simulink model "exercise_5_1"  (R2024a)
settings: Solver=VariableStepDiscrete  StartTime=0.0  StopTime=inf  RelTol=1e-3  EnableMultiTasking=on
libraries: simulink_extras x3
settings Model: Creator=nunkesser  LastModifiedBy=nunkesser
settings SolverCC: AlgebraicLoopSolver=TrustRegion
settings DataIOCC: LimitDataPoints=on  SaveFormat=Array  ReturnWorkspaceOutputs=off
settings OptimizationCC: LifeSpan=inf
settings DebuggingCC: SolverPrmCheckMsg=warning  UnconnectedInputMsg=warning  UnconnectedOutputMsg=warning  UnconnectedLineMsg=warning  AllowSymbolicDim=off  SFUnexpectedBacktrackingDiag=warning  SFNoUnconditionalDefaultTransitionDiag=warning  SFExecutionAtInitializationDiag=none  ArithmeticOperatorsInVariantConditions=warning
settings HardwareCC: ProdBitPerPointer=32  ProdBitPerSizeT=32  ProdBitPerPtrDiffT=32  ProdLargestAtomicFloat=None  ProdIntDivRoundTo=Undefined  ProdEndianess=Unspecified  ProdWordSize=32  ProdHWDeviceType=32-bit Generic
settings ModelReferenceCC: EnableRefExpFcnMdlSchedulingChecks=on  PropagateSignalLabelsOutOfModel=off
settings SFSimCC: SimUseLocalCustomCode=off  CustomCodeUndefinedFunction=UseInterfaceOnly
settings RTWCC: RTWUseLocalCustomCode=off  GPUComputeCapability=3.5
settings CodeAppCC: StateflowObjectComments=on
settings GRTTargetCC: TargetLangStandard=C89/C90 (ANSI)
settings ConfigComp: CovMetricSettings=dw  CovSaveCumulativeToWorkspaceVar=on  CovSaveSingleToWorkspaceVar=on  CovExternalEMLEnable=off  CovSFcnEnable=off

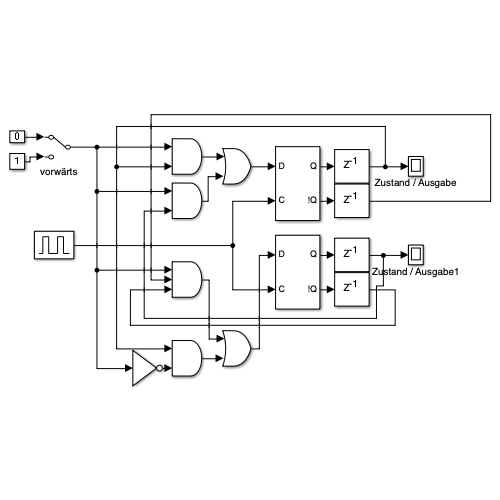
[thumbnail: Simulink's stored preview of the top-level diagram]
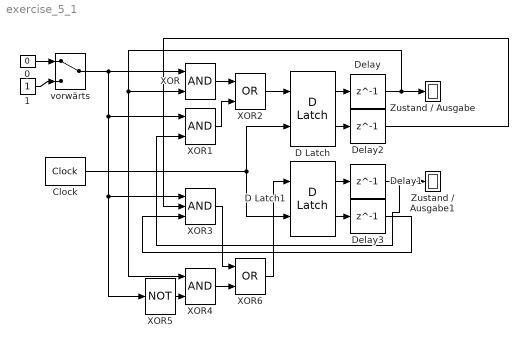
== system exercise_5_1 ==
  "0 " : Constant  Value=0  OutDataTypeStr=boolean
  1 : Constant  OutDataTypeStr=boolean
  Clock : simulink_extras/Flip Flops/Clock  period=2
  D Latch : simulink_extras/Flip Flops/D Latch
  D Latch1 : simulink_extras/Flip Flops/D Latch
  Delay{,1..3} (4 alike) : Delay  DelayLength=1  InitialCondition=0  SampleTime=1
  XOR : Logic  IconShape=distinctive  OutDataTypeStr=boolean
  XOR1 : Logic  IconShape=distinctive  OutDataTypeStr=boolean
  XOR2 : Logic  Operator=OR  IconShape=distinctive  OutDataTypeStr=boolean
  XOR3 : Logic  Inputs=3  IconShape=distinctive  OutDataTypeStr=boolean
  XOR4 : Logic  IconShape=distinctive  OutDataTypeStr=boolean
  XOR5 : Logic  Operator=NOT  IconShape=distinctive  OutDataTypeStr=boolean
  XOR6 : Logic  Operator=OR  IconShape=distinctive  OutDataTypeStr=boolean
  Zustand / Ausgabe : Display
  Zustand / Ausgabe1 : Display
  vorwärts : ManualSwitch
  wires:
  XOR/1 -> XOR2/1
  1/1 -> vorwärts/2
  "0 "/1 -> vorwärts/1
  vorwärts/1 -> XOR/1, XOR1/1, XOR5/1, XOR3/1
  D Latch/1 -> Delay/1
  Delay/1 -> XOR/2, XOR4/1, Zustand / Ausgabe/1
  Clock/1 -> D Latch1/2, D Latch/2
  D Latch1/1 -> Delay1/1
  Delay1/1 -> Zustand / Ausgabe1/1, XOR1/2
  XOR2/1 -> D Latch/1
  XOR1/1 -> XOR2/2
  D Latch/2 -> Delay2/1
  D Latch1/2 -> Delay3/1
  Delay3/1 -> XOR3/3
  Delay2/1 -> XOR3/2
  XOR5/1 -> XOR4/2
  XOR6/1 -> D Latch1/1
  XOR3/1 -> XOR6/1
  XOR4/1 -> XOR6/2
